simulink model "Visualization"  (R2020a)
settings: Solver=VariableStepAuto  StartTime=0.0  StopTime=10.0  RelTol=1e-3
model workspace (MAT data in the model file):
  VEH.Mass = 330
  VEH.StaticNormalFrontLoad.FR = 74.25
  VEH.StaticNormalFrontLoad.FL = 74.25
  VEH.StaticNormalRearLoad.RR = 90.75
  VEH.StaticNormalRearLoad.RL = 90.75
  VEH.WheelBase = 1.54
  VEH.FrontAxlePositionfromCG = 0.847
  VEH.RearAxlePositionfromCG = 0.693
  VEH.HeightCG = 0.283
  VEH.FrontalArea = 2.11
  VEH.DragCoefficient = 0.33
  VEH.NumberOfWheelsPerAxle = 2
  VEH.Thread.FR = 1.705
  VEH.Thread.RR = 1.705
  VEH.PitchMomentInertia = 206
  VEH.RollMomentInertia = 206.613792
  VEH.YawMomentInertia = 206.613792
  VEH.SteeringRatio = 5.2
  VEH.TrackWidth = 1.2
  VEH.SprungMass = 290
  VEH.InitialLongPosition = 0
  VEH.InitialLatPosition = 0
  VEH.InitialVertPosition = 0
  VEH.InitialRollAngle = 0
  VEH.InitialPitchAngle = 0
  VEH.InitialYawAngle = 0
  VEH.InitialLongVel = 0
  VEH.InitialLatVel = 0
  VEH.InitialVertVel = 0
  VEH.InitialRollRate = 0
  VEH.InitialPitchRate = 0
  VEH.InitialYawRate = 0
undefined symbols (not defined in the file): h
libraries: sim3dlib x2, simulink x1, vehdynlibviscommon x1
settings Model: Creator=Administrator  LastModifiedBy=Administrator

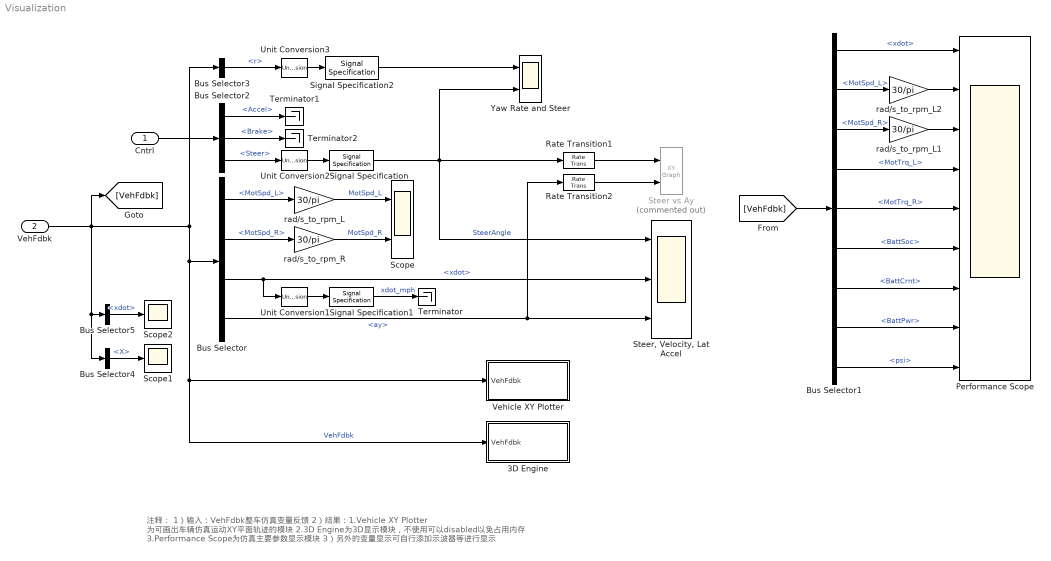
== system Visualization ==
  note: 注释：
      | 1）输入：VehFdbk整车仿真变量反馈
      | 2）结果：1.Vehicle XY Plotter 为可画出车辆仿真运动XY平面轨迹的模块
      | 2.3D Engine为3D显示模块，不使用可以disabled以免占用内存
      | 3.Performance Scope为仿真主要参数显示模块
      | 3）另外的变量显示可自行添加示波器等进行显示
  Cntrl : Inport
  VehFdbk : Inport  Port=2
  3D Engine : Subsystem  Variant=on  VariantControlMode=Label  LabelModeActiveChoice=0  mask(3D Engine){engine3D=Disabled, SceneDesc=Straight road, dt3D=.03}
      mask prompts: engine3D "3D Engine"; SceneDesc "Scene Description:"; dt3D "Engine frame rate, dt3D [s]:"
      mask help: This subsystem contains the interface blocks which permit the display of the vehicle in 3D virtual environment. Enable it to view the simulation progress, disable it to inhibit the display.
      mask init:
      | switch get_param(gcb,'engine3D')
      |     case 'Disabled'
      |         set_param(gcb,'OverrideUsingVariant','0')
      |     case 'Enabled'
      |        set_param(gcb,'OverrideUsingVariant','1')
      |     otherwise
      |        set_param(gcb,'OverrideUsingVariant','0')
      | end
      settings: AttributesFormatString=%<engine3D>
      mask Help: eval('vdynblkshelp(''vdynblksscenecameraray'')');
      mask TypeOptions engine3D: Enabled | Disabled
      mask Callback engine3D:
      | switch get_param(gcb,'engine3D')
      |     case 'Disabled'
      |         set_param(gcb,'OverrideUsingVariant','0')
      |     case 'Enabled'
      |        set_param(gcb,'OverrideUsingVariant','1')
      |     otherwise
      |        set_param(gcb,'OverrideUsingVariant','0')
      | end
      mask TypeOptions SceneDesc:
      | 3D Engine/Simulation 3D Engine
      | 1/SceneDesc
      mask Display: disp('3D Engine')
  Bus Selector : BusSelector  OutputSignals=MotSpd_L,MotSpd_R,Body.xdot,Body.ay
  Bus Selector1 : BusSelector  OutputSignals=Body.xdot,MotSpd_L,MotSpd_R,ElecFdbk.MotTrq_L,ElecFdbk.MotTrq_R,ElecFdbk.BattSoc,ElecFdbk.BattCrnt,ElecFdbk.BattPwr,Body.psi
  Bus Selector2 : BusSelector  OutputSignals=Accel,Brake,Steer
  Bus Selector3 : BusSelector  OutputSignals=Body.r
  Bus Selector4 : BusSelector  OutputSignals=Body.X
  Bus Selector5 : BusSelector  OutputSignals=Body.xdot
  Performance Scope : Scope  NumInputPorts=9
  Rate Transition1 : RateTransition  OutPortSampleTime=.1
  Rate Transition2 : RateTransition  OutPortSampleTime=.1
  Scope : Scope  NumInputPorts=2
  Scope1 : Scope
  Scope2 : Scope
  Signal Specification : SignalSpecification  Unit=deg
  Signal Specification1 : SignalSpecification  Unit=mph
  Signal Specification2 : SignalSpecification  Unit=deg/s
  Steer vs Ay : simulink/Sinks/XY Graph  Commented=on  xmin=-300  xmax=300  ymin=-1.5  ymax=1.5  st=.1
  "Steer, Velocity, Lat Accel" : Scope  NumInputPorts=3
  Terminator : Terminator
  Terminator1 : Terminator
  Terminator2 : Terminator
  Unit Conversion1 : UnitConversion
  Unit Conversion2 : UnitConversion
  Unit Conversion3 : UnitConversion
  Vehicle XY Plotter : Subsystem  mask(Vehicle XY Plotter){a=VEH.FrontAxlePositionfromCG, b=VEH.RearAxlePositionfromCG, w=VEH.TrackWidth, bufferSize=1024, pltDT=.1}
      mask prompts: a "Distance to front axle from CG, a [m]:"; b "Distance to rear axle from CG, b [m]:"; w "Track width, w [m]:"; bufferSize "Path buffer sampe size, bufferSize []:"; pltDT "Plot update rate, pltDT [s]:"
      mask help: This block will display a MATLAB figure which indicates the vehicle path, current position and heading velocity.
      mask TypeOptions a: Vehicle XY Plotter/a
      mask TypeOptions b: Vehicle XY Plotter/b
      mask TypeOptions w: Vehicle XY Plotter/w
      mask TypeOptions bufferSize: Vehicle XY Plotter/bufferSize
  Yaw Rate and Steer : Scope  NumInputPorts=2
  rad/s_to_rpm_L : Gain  Gain=30/pi
  rad/s_to_rpm_L1 : Gain  Gain=30/pi
  rad/s_to_rpm_L2 : Gain  Gain=30/pi
  rad/s_to_rpm_R : Gain  Gain=30/pi
  wires:
  Bus Selector2/1 -> Terminator1/1  "<Accel>"
  rad/s_to_rpm_R/1 -> Scope/2  "MotSpd_R"
  Bus Selector1/3 -> rad/s_to_rpm_L1/1  "<MotSpd_R>"
  rad/s_to_rpm_L1/1 -> Performance Scope/3
  Signal Specification1/1 -> Terminator/1  "xdot_mph"
  Bus Selector/3 -> Unit Conversion1/1, "Steer, Velocity, Lat Accel"/2  "<xdot>"
  Bus Selector1/4 -> Performance Scope/4  "<MotTrq_L>"
  Bus Selector2/3 -> Unit Conversion2/1  "<Steer>"
  rad/s_to_rpm_L2/1 -> Performance Scope/2
  Bus Selector1/2 -> rad/s_to_rpm_L2/1  "<MotSpd_L>"
  Bus Selector1/6 -> Performance Scope/6  "<BattSoc>"
  Unit Conversion1/1 -> Signal Specification1/1
  [VehFdbk] -> Bus Selector1/1
  Signal Specification/1 -> Yaw Rate and Steer/2, Rate Transition1/1, "Steer, Velocity, Lat Accel"/1  "SteerAngle"
  Bus Selector1/5 -> Performance Scope/5  "<MotTrq_R>"
  VehFdbk/1 -> Bus Selector5/1, Bus Selector4/1, [VehFdbk], Bus Selector/1, Vehicle XY Plotter/1(VehFdbk), 3D Engine/1(VehFdbk), Bus Selector3/1  "VehFdbk"
  Bus Selector2/2 -> Terminator2/1  "<Brake>"
  Bus Selector1/1 -> Performance Scope/1  "<xdot>"
  Bus Selector4/1 -> Scope1/1  "<X>"
  Bus Selector1/7 -> Performance Scope/7  "<BattCrnt>"
  Bus Selector1/8 -> Performance Scope/8  "<BattPwr>"
  Rate Transition1/1 -> Steer vs Ay/1
  Bus Selector/4 -> Rate Transition2/1, "Steer, Velocity, Lat Accel"/3  "<ay>"
  Cntrl/1 -> Bus Selector2/1
  Unit Conversion3/1 -> Signal Specification2/1
  Bus Selector/1 -> rad/s_to_rpm_L/1  "<MotSpd_L>"
  Bus Selector3/1 -> Unit Conversion3/1  "<r>"
  Unit Conversion2/1 -> Signal Specification/1
  Rate Transition2/1 -> Steer vs Ay/2
  Bus Selector5/1 -> Scope2/1  "<xdot>"
  rad/s_to_rpm_L/1 -> Scope/1  "MotSpd_L"
  Signal Specification2/1 -> Yaw Rate and Steer/1
  Bus Selector/2 -> rad/s_to_rpm_R/1  "<MotSpd_R>"
  Bus Selector1/9 -> Performance Scope/9  "<psi>"

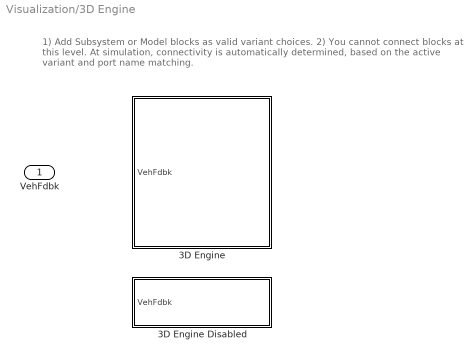
== system Visualization/3D Engine ==
  note: 1) Add Subsystem or Model blocks as valid variant choices.
      | 2) You cannot connect blocks at this level. At simulation, connectivity is automatically
      | determined, based on the active variant and port name matching.
  VehFdbk : Inport
  3D Engine : Subsystem  VariantControl=1
  3D Engine Disabled : Subsystem  VariantControl=0

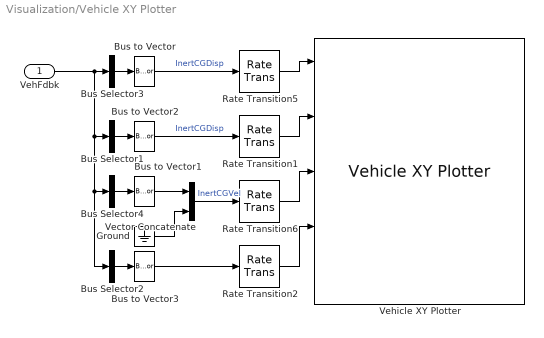
== system Visualization/Vehicle XY Plotter ==
  VehFdbk : Inport
  Bus Selector1 : BusSelector  OutputSignals=Body.phi,Body.theta,Body.psi  OutputAsBus=on
  Bus Selector2 : BusSelector  OutputSignals=Driveline.WhlAng  OutputAsBus=on
  Bus Selector3 : BusSelector  OutputSignals=Body.X,Body.Y,Body.Z  OutputAsBus=on
  Bus Selector4 : BusSelector  OutputSignals=Body.Xdot,Body.Ydot  OutputAsBus=on
  Bus to Vector{,1..3} (4 alike) : BusToVector
  Ground : Ground
  Rate Transition{1..2,5..6} (4 alike) : RateTransition  OutPortSampleTime=pltDT
  Vector Concatenate : Concatenate
  Vehicle XY Plotter : vehdynlibviscommon/Vehicle XY Plotter  bufferSize=bufferSize  w=w  a=a  b=b  figBorder=1
      settings: SourceProductBaseCode=VE
  wires:
  Bus to Vector2/1 -> Rate Transition1/1  "InertCGDisp"
  Rate Transition5/1 -> Vehicle XY Plotter/1
  Bus Selector4/1 -> Bus to Vector1/1
  Rate Transition1/1 -> Vehicle XY Plotter/2
  Rate Transition6/1 -> Vehicle XY Plotter/3
  Vector Concatenate/1 -> Rate Transition6/1  "InertCGVel"
  Bus Selector1/1 -> Bus to Vector2/1
  Bus to Vector/1 -> Rate Transition5/1  "InertCGDisp"
  Bus Selector3/1 -> Bus to Vector/1
  Bus to Vector1/1 -> Vector Concatenate/1
  Ground/1 -> Vector Concatenate/2
  Bus to Vector3/1 -> Rate Transition2/1
  Bus Selector2/1 -> Bus to Vector3/1
  VehFdbk/1 -> Bus Selector1/1, Bus Selector2/1, Bus Selector4/1, Bus Selector3/1
  Rate Transition2/1 -> Vehicle XY Plotter/4

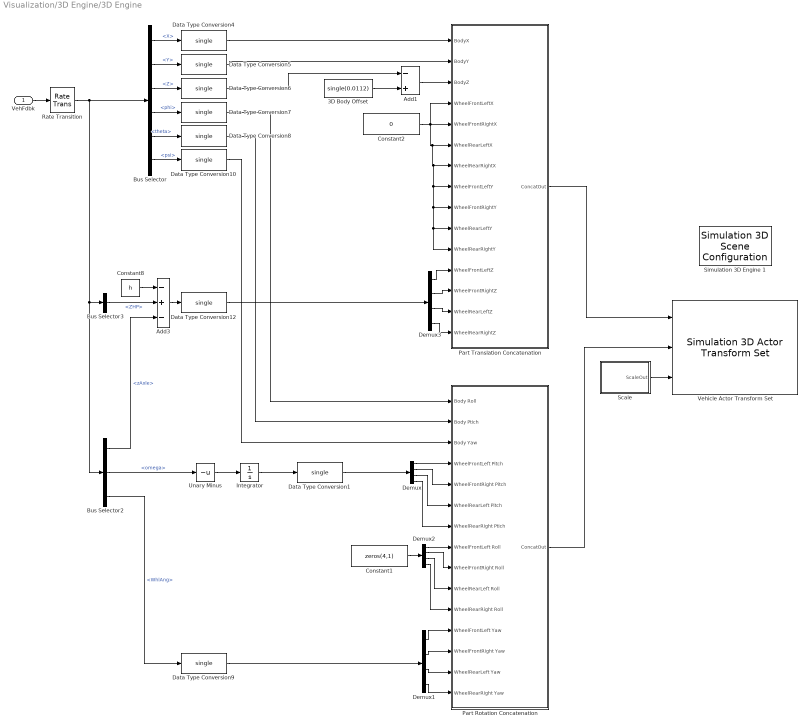
== system Visualization/3D Engine/3D Engine ==
  VehFdbk : Inport
  3D Body Offset : Constant  Value=single(0.0112)  OutDataTypeStr=single
  Add1 : Sum  Inputs=-+
  Add3 : Sum  Inputs=-+-
  Bus Selector : BusSelector  OutputSignals=Body.X,Body.Y,Body.Z,Body.phi,Body.theta,Body.psi
  Bus Selector2 : BusSelector  OutputSignals=Wheels.zAxle,Wheels.omega,Driveline.WhlAng
  Bus Selector3 : BusSelector  OutputSignals=Body.ZHP
  Constant1 : Constant  Value=zeros(4,1)  OutDataTypeStr=single
  Constant2 : Constant  Value=0  OutDataTypeStr=single
  Constant8 : Constant  Value=h
  Data Type Conversion{1,4..10,12} (9 alike) : DataTypeConversion  OutDataTypeStr=single
  Demux{,1..3} (4 alike) : Demux
  Integrator : Integrator  WrapState=on  WrappedStateUpperValue=2*pi  WrappedStateLowerValue=0  ZeroCross=off
  Part Rotation Concatenation : Subsystem
  Part Translation Concatenation : Subsystem
  Rate Transition : RateTransition  OutPortSampleTime=dt3D
  Scale : Subsystem
  Simulation 3D Engine 1 : sim3dlib/Simulation 3D Scene Configuration  Priority=1  ProjectFormat=Default Scenes  SceneDesc=Straight road  ProjectName=VehicleSimulation.exe  ScenePath=/Game/Maps/HwStrght  vehTagList={'Scene Origin'}  vehTag=Scene Origin  OpVisEn=off  Ts=dt3D  EnableWindow=on  sensorTag=MainCamera1  sensorId=1  sensorName=MainCamera1  mountLoc=Origin  offsetFlag=off  tmountOffset=[0, 0, 0]  rmountOffset=[0, 0, 0]  HorizontalResolution=1280  VerticalResolution=720  HorizontalFOV=60  mountPoint=[0 0 0]  mountOrientation=[0 0 0]  aMode=aMode  ID=1
      settings: AttributesFormatString=Priority: %<Priority>  SourceProductBaseCode=DR,VE
  Unary Minus : UnaryMinus
  Vehicle Actor Transform Set : sim3dlib/Simulation 3D Actor Transform Set  ActorTag=SimulinkVehicle1  ActorType=Passenger vehicle  PassVehMesh=Muscle car  VehColor=Red  NumberOfParts=5  CustNumOfParts=3  Translation=[0 0 1; 0 0 0; 0 0 0; 0 0 0; 0 0 0]  Rotation=[0 0 0; 0 0 0; 0 0 0; 0 0 0; 0 0 0]  Scale=[1 1 1; 1 1 1; 1 1 1; 1 1 1; 1 1 1]  Ts=dt3D
      settings: SourceProductBaseCode=DR,VE
  wires:
  Unary Minus/1 -> Integrator/1
  Bus Selector3/1 -> Add3/2  "<ZHP>"
  Add3/1 -> Data Type Conversion12/1
  Bus Selector2/1 -> Add3/3  "<zAxle>"
  Constant8/1 -> Add3/1
  Rate Transition/1 -> Bus Selector/1, Bus Selector3/1, Bus Selector2/1
  Scale/1(ScaleOut) -> Vehicle Actor Transform Set/3
  Demux/4 -> Part Rotation Concatenation/7(WheelRearRight Ptich)
  Demux/3 -> Part Rotation Concatenation/6(WheelRearLeft Pitch)
  Demux/2 -> Part Rotation Concatenation/5(WheelFrontRight Pitch)
  Demux/1 -> Part Rotation Concatenation/4(WheelFrontLeft Pitch)
  Constant1/1 -> Demux2/1
  Bus Selector/4 -> Data Type Conversion7/1  "<phi>"
  Data Type Conversion6/1 -> Add1/1
  Part Rotation Concatenation/1(ConcatOut) -> Vehicle Actor Transform Set/2
  Part Translation Concatenation/1(ConcatOut) -> Vehicle Actor Transform Set/1
  Data Type Conversion12/1 -> Demux3/1
  Demux3/4 -> Part Translation Concatenation/15(WheelRearRightZ)
  Demux3/3 -> Part Translation Concatenation/14(WheelRearLeftZ)
  Demux3/1 -> Part Translation Concatenation/12(WheelFrontLeftZ)
  Demux3/2 -> Part Translation Concatenation/13(WheelFrontRightZ)
  VehFdbk/1 -> Rate Transition/1
  Add1/1 -> Part Translation Concatenation/3(BodyZ)
  3D Body Offset/1 -> Add1/2
  Demux1/4 -> Part Rotation Concatenation/15(WheelRearRight Yaw)
  Demux1/3 -> Part Rotation Concatenation/14(WheelRearLeft Yaw)
  Demux2/1 -> Part Rotation Concatenation/8(WheelFrontLeft Roll)
  Demux2/2 -> Part Rotation Concatenation/9(WheelFrontRight Roll)
  Demux2/3 -> Part Rotation Concatenation/10(WheelRearLeft Roll)
  Demux2/4 -> Part Rotation Concatenation/11(WheelRearRight Roll)
  Bus Selector2/3 -> Data Type Conversion9/1  "<WhlAng>"
  Bus Selector2/2 -> Unary Minus/1  "<omega>"
  Data Type Conversion9/1 -> Demux1/1
  Demux1/1 -> Part Rotation Concatenation/12(WheelFrontLeft Yaw)
  Demux1/2 -> Part Rotation Concatenation/13(WheelFrontRight Yaw)
  Integrator/1 -> Data Type Conversion1/1
  Data Type Conversion1/1 -> Demux/1
  Data Type Conversion8/1 -> Part Rotation Concatenation/2(Body Ptich)
  Data Type Conversion5/1 -> Part Translation Concatenation/2(BodyY)
  Data Type Conversion10/1 -> Part Rotation Concatenation/3(Body Yaw)
  Constant2/1 -> Part Translation Concatenation/5(WheelFrontRightX), Part Translation Concatenation/6(WheelRearLeftX), Part Translation Concatenation/7(WheelRearRightX), Part Translation Concatenation/8(WheelFrontLeftY), Part Translation Concatenation/9(WheelFrontRightY), Part Translation Concatenation/10(WheelRearLeftY), Part Translation Concatenation/11(WheelRearRightY), Part Translation Concatenation/4(WheelFrontLeftX)
  Data Type Conversion4/1 -> Part Translation Concatenation/1(BodyX)
  Data Type Conversion7/1 -> Part Rotation Concatenation/1(Body Roll)
  Bus Selector/1 -> Data Type Conversion4/1  "<X>"
  Bus Selector/2 -> Data Type Conversion5/1  "<Y>"
  Bus Selector/3 -> Data Type Conversion6/1  "<Z>"
  Bus Selector/6 -> Data Type Conversion10/1  "<psi>"
  Bus Selector/5 -> Data Type Conversion8/1  "<theta>"

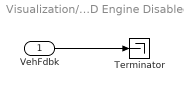
== system Visualization/3D Engine/3D Engine Disabled ==
  VehFdbk : Inport
  Terminator : Terminator
  wires:
  VehFdbk/1 -> Terminator/1

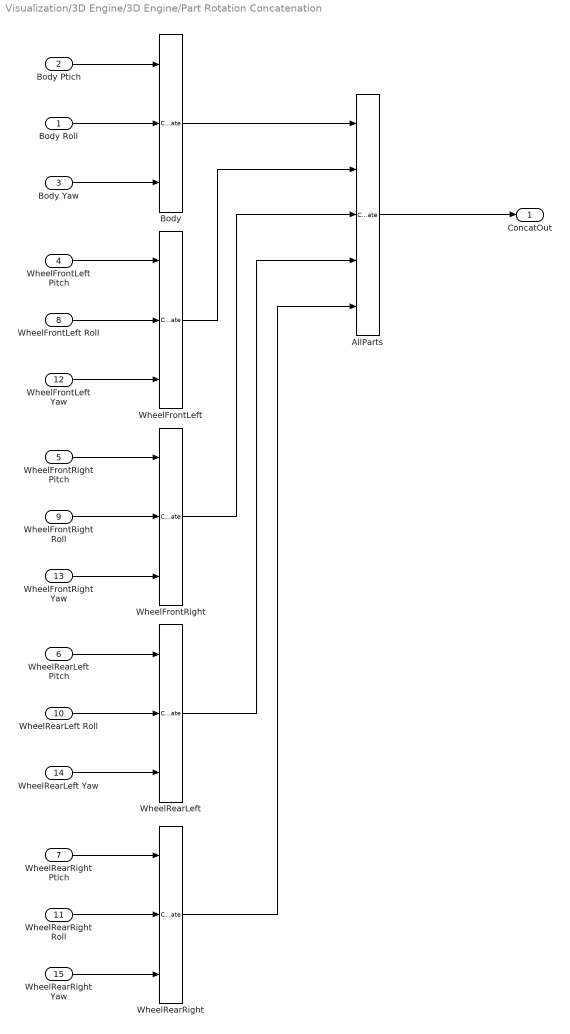
== system Visualization/3D Engine/3D Engine/Part Rotation Concatenation ==
  Body Roll : Inport
  Body Ptich : Inport  Port=2
  Body Yaw : Inport  Port=3
  WheelFrontLeft Pitch : Inport  Port=4
  WheelFrontRight Pitch : Inport  Port=5
  WheelRearLeft Pitch : Inport  Port=6
  WheelRearRight Ptich : Inport  Port=7
  WheelFrontLeft Roll : Inport  Port=8
  WheelFrontRight Roll : Inport  Port=9
  WheelRearLeft Roll : Inport  Port=10
  WheelRearRight Roll : Inport  Port=11
  WheelFrontLeft Yaw : Inport  Port=12
  WheelFrontRight Yaw : Inport  Port=13
  WheelRearLeft Yaw : Inport  Port=14
  WheelRearRight Yaw : Inport  Port=15
  AllParts : Concatenate  NumInputs=5  Mode=Multidimensional array
  Body : Concatenate  NumInputs=3  Mode=Multidimensional array  ConcatenateDimension=2
  WheelFrontLeft : Concatenate  NumInputs=3  Mode=Multidimensional array  ConcatenateDimension=2
  WheelFrontRight : Concatenate  NumInputs=3  Mode=Multidimensional array  ConcatenateDimension=2
  WheelRearLeft : Concatenate  NumInputs=3  Mode=Multidimensional array  ConcatenateDimension=2
  WheelRearRight : Concatenate  NumInputs=3  Mode=Multidimensional array  ConcatenateDimension=2
  ConcatOut : Outport  VectorParamsAs1DForOutWhenUnconnected=off
  wires:
  Body Ptich/1 -> Body/1
  Body Yaw/1 -> Body/3
  WheelFrontLeft Pitch/1 -> WheelFrontLeft/1
  WheelFrontLeft Yaw/1 -> WheelFrontLeft/3
  WheelFrontLeft Roll/1 -> WheelFrontLeft/2
  Body Roll/1 -> Body/2
  WheelFrontLeft/1 -> AllParts/2
  WheelRearRight Ptich/1 -> WheelRearRight/1
  Body/1 -> AllParts/1
  WheelRearLeft/1 -> AllParts/4
  WheelFrontRight/1 -> AllParts/3
  WheelRearRight Yaw/1 -> WheelRearRight/3
  WheelFrontRight Roll/1 -> WheelFrontRight/2
  WheelFrontRight Pitch/1 -> WheelFrontRight/1
  WheelRearRight Roll/1 -> WheelRearRight/2
  WheelRearLeft Yaw/1 -> WheelRearLeft/3
  AllParts/1 -> ConcatOut/1
  WheelRearLeft Roll/1 -> WheelRearLeft/2
  WheelRearRight/1 -> AllParts/5
  WheelRearLeft Pitch/1 -> WheelRearLeft/1
  WheelFrontRight Yaw/1 -> WheelFrontRight/3

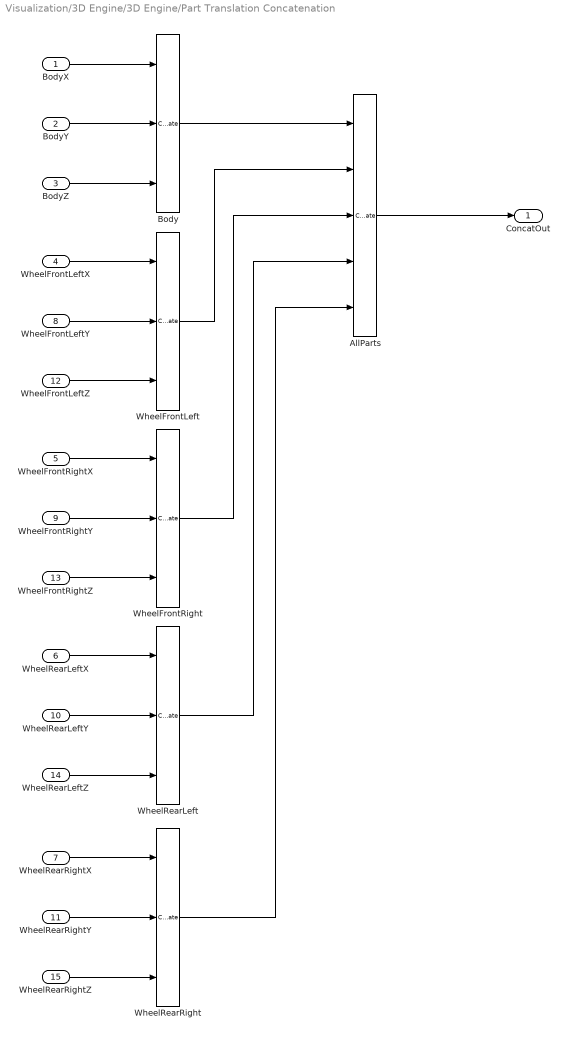
== system Visualization/3D Engine/3D Engine/Part Translation Concatenation ==
  BodyX : Inport
  BodyY : Inport  Port=2
  BodyZ : Inport  Port=3
  WheelFrontLeftX : Inport  Port=4
  WheelFrontRightX : Inport  Port=5
  WheelRearLeftX : Inport  Port=6
  WheelRearRightX : Inport  Port=7
  WheelFrontLeftY : Inport  Port=8
  WheelFrontRightY : Inport  Port=9
  WheelRearLeftY : Inport  Port=10
  WheelRearRightY : Inport  Port=11
  WheelFrontLeftZ : Inport  Port=12
  WheelFrontRightZ : Inport  Port=13
  WheelRearLeftZ : Inport  Port=14
  WheelRearRightZ : Inport  Port=15
  AllParts : Concatenate  NumInputs=5  Mode=Multidimensional array
  Body : Concatenate  NumInputs=3  Mode=Multidimensional array  ConcatenateDimension=2
  WheelFrontLeft : Concatenate  NumInputs=3  Mode=Multidimensional array  ConcatenateDimension=2
  WheelFrontRight : Concatenate  NumInputs=3  Mode=Multidimensional array  ConcatenateDimension=2
  WheelRearLeft : Concatenate  NumInputs=3  Mode=Multidimensional array  ConcatenateDimension=2
  WheelRearRight : Concatenate  NumInputs=3  Mode=Multidimensional array  ConcatenateDimension=2
  ConcatOut : Outport  VectorParamsAs1DForOutWhenUnconnected=off
  wires:
  BodyX/1 -> Body/1
  BodyZ/1 -> Body/3
  WheelFrontLeftX/1 -> WheelFrontLeft/1
  WheelFrontLeftZ/1 -> WheelFrontLeft/3
  WheelFrontLeftY/1 -> WheelFrontLeft/2
  BodyY/1 -> Body/2
  WheelFrontLeft/1 -> AllParts/2
  WheelRearRightX/1 -> WheelRearRight/1
  Body/1 -> AllParts/1
  WheelRearLeft/1 -> AllParts/4
  WheelFrontRight/1 -> AllParts/3
  WheelRearRightZ/1 -> WheelRearRight/3
  WheelFrontRightY/1 -> WheelFrontRight/2
  WheelFrontRightX/1 -> WheelFrontRight/1
  WheelRearRightY/1 -> WheelRearRight/2
  WheelRearLeftZ/1 -> WheelRearLeft/3
  AllParts/1 -> ConcatOut/1
  WheelRearLeftY/1 -> WheelRearLeft/2
  WheelRearRight/1 -> AllParts/5
  WheelRearLeftX/1 -> WheelRearLeft/1
  WheelFrontRightZ/1 -> WheelFrontRight/3

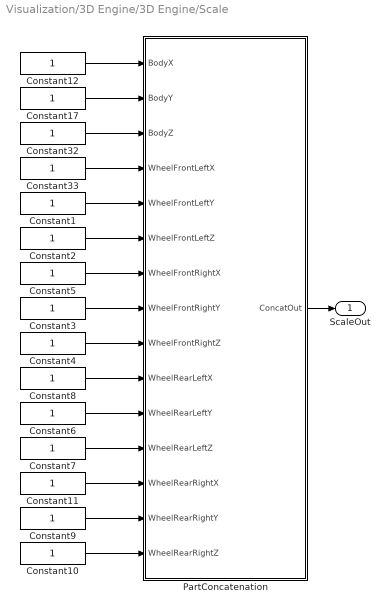
== system Visualization/3D Engine/3D Engine/Scale ==
  Constant{1..12,17,32..33} (15 alike) : Constant  OutDataTypeStr=single
  PartConcatenation : Subsystem
  ScaleOut : Outport  VectorParamsAs1DForOutWhenUnconnected=off
  wires:
  Constant10/1 -> PartConcatenation/15(WheelRearRightZ)
  Constant9/1 -> PartConcatenation/14(WheelRearRightY)
  Constant11/1 -> PartConcatenation/13(WheelRearRightX)
  Constant7/1 -> PartConcatenation/12(WheelRearLeftZ)
  Constant6/1 -> PartConcatenation/11(WheelRearLeftY)
  Constant8/1 -> PartConcatenation/10(WheelRearLeftX)
  Constant4/1 -> PartConcatenation/9(WheelFrontRightZ)
  Constant3/1 -> PartConcatenation/8(WheelFrontRightY)
  Constant5/1 -> PartConcatenation/7(WheelFrontRightX)
  Constant2/1 -> PartConcatenation/6(WheelFrontLeftZ)
  Constant1/1 -> PartConcatenation/5(WheelFrontLeftY)
  Constant33/1 -> PartConcatenation/4(WheelFrontLeftX)
  Constant32/1 -> PartConcatenation/3(BodyZ)
  Constant17/1 -> PartConcatenation/2(BodyY)
  Constant12/1 -> PartConcatenation/1(BodyX)
  PartConcatenation/1(ConcatOut) -> ScaleOut/1

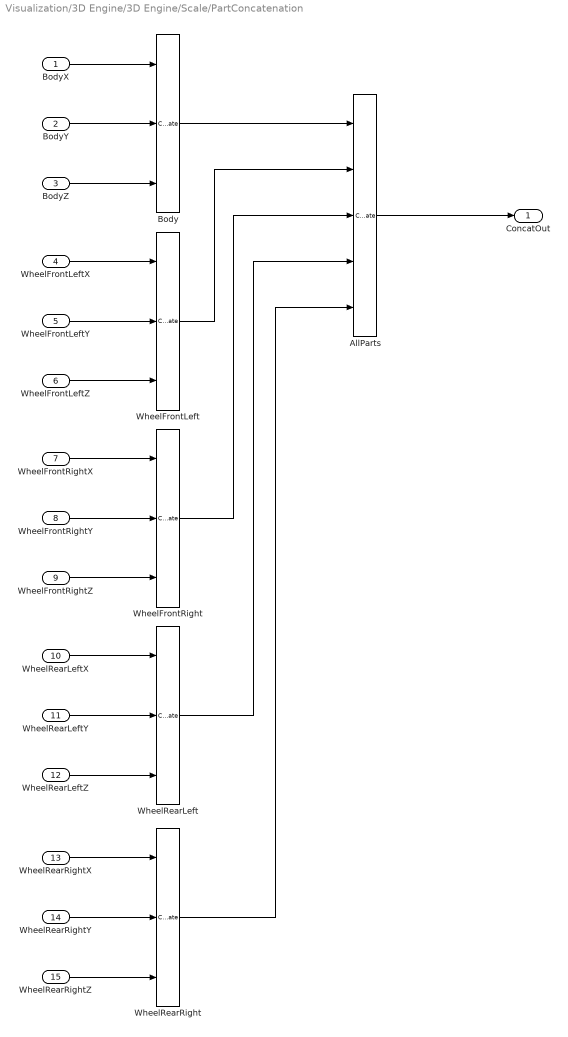
== system Visualization/3D Engine/3D Engine/Scale/PartConcatenation ==
  BodyX : Inport
  BodyY : Inport  Port=2
  BodyZ : Inport  Port=3
  WheelFrontLeftX : Inport  Port=4
  WheelFrontLeftY : Inport  Port=5
  WheelFrontLeftZ : Inport  Port=6
  WheelFrontRightX : Inport  Port=7
  WheelFrontRightY : Inport  Port=8
  WheelFrontRightZ : Inport  Port=9
  WheelRearLeftX : Inport  Port=10
  WheelRearLeftY : Inport  Port=11
  WheelRearLeftZ : Inport  Port=12
  WheelRearRightX : Inport  Port=13
  WheelRearRightY : Inport  Port=14
  WheelRearRightZ : Inport  Port=15
  AllParts : Concatenate  NumInputs=5  Mode=Multidimensional array
  Body : Concatenate  NumInputs=3  Mode=Multidimensional array  ConcatenateDimension=2
  WheelFrontLeft : Concatenate  NumInputs=3  Mode=Multidimensional array  ConcatenateDimension=2
  WheelFrontRight : Concatenate  NumInputs=3  Mode=Multidimensional array  ConcatenateDimension=2
  WheelRearLeft : Concatenate  NumInputs=3  Mode=Multidimensional array  ConcatenateDimension=2
  WheelRearRight : Concatenate  NumInputs=3  Mode=Multidimensional array  ConcatenateDimension=2
  ConcatOut : Outport  VectorParamsAs1DForOutWhenUnconnected=off
  wires:
  BodyX/1 -> Body/1
  BodyZ/1 -> Body/3
  WheelFrontLeftX/1 -> WheelFrontLeft/1
  WheelFrontLeftZ/1 -> WheelFrontLeft/3
  WheelFrontLeftY/1 -> WheelFrontLeft/2
  BodyY/1 -> Body/2
  WheelFrontLeft/1 -> AllParts/2
  WheelRearRightX/1 -> WheelRearRight/1
  Body/1 -> AllParts/1
  WheelRearLeft/1 -> AllParts/4
  WheelFrontRight/1 -> AllParts/3
  WheelRearRightZ/1 -> WheelRearRight/3
  WheelFrontRightY/1 -> WheelFrontRight/2
  WheelFrontRightX/1 -> WheelFrontRight/1
  WheelRearRightY/1 -> WheelRearRight/2
  WheelRearLeftZ/1 -> WheelRearLeft/3
  AllParts/1 -> ConcatOut/1
  WheelRearLeftY/1 -> WheelRearLeft/2
  WheelRearRight/1 -> AllParts/5
  WheelRearLeftX/1 -> WheelRearLeft/1
  WheelFrontRightZ/1 -> WheelFrontRight/3
